simulink model "NeuromuscularModel3D"  (R2019b)
settings: Solver=ode15s  StartTime=0.0  StopTime=30  MaxStep=.01  RelTol=1e-4  AbsTol=1e-6  EnableMultiTasking=on
values from neighbouring files (symbols this model uses):
  dt_visual = 1/1000    (= 0.001)    [demorun.m]    (also in evaluateCost.m = 0.0333333333333; optimize.m = 0.0333333333333; optimize_Conly.m = 0.0333333333333; setVars.m = 0.0333333333333)
  initialTargetAngle = 70*pi/180    (= 1.2217304764)    [setInit.m]
  initialTargetAngleR = 90*pi/180    (= 1.57079632679)    [setInit.m]
  LongDelay = 0.020    (= 0.02)    [ControlParams2.m]
  MidDelay = 0.010    (= 0.01)    [ControlParams2.m]
  N = 82    [vcmaes_1.5cm_0.9ms_Umb10_kneelim1_mstoptorque2.mat]
  PreStimBFSHst = Gains(66)    [assignGains.m]    (also in assignGainsSagittal.m = GainsSagittal(51))
  PreStimBFSHsw = Gains(77)    [assignGains.m]    (also in assignGainsSagittal.m = GainsSagittal(60))
  PreStimGASst = Gains(67)    [assignGains.m]    (also in assignGainsSagittal.m = GainsSagittal(52))
  PreStimGASsw = Gains(78)    [assignGains.m]    (also in assignGainsSagittal.m = GainsSagittal(61))
  PreStimGLUst = Gains(62)    [assignGains.m]    (also in assignGainsSagittal.m = GainsSagittal(47))
  PreStimGLUsw = Gains(73)    [assignGains.m]    (also in assignGainsSagittal.m = GainsSagittal(56))
  PreStimHABst = Gains(70)    [assignGains.m]    (also in assignGainsCoronal.m = GainsCoronal(15))
  PreStimHABsw = Gains(81)    [assignGains.m]    (also in assignGainsCoronal.m = GainsCoronal(17))
  PreStimHADst = Gains(71)    [assignGains.m]    (also in assignGainsCoronal.m = GainsCoronal(16))
  PreStimHADsw = Gains(82)    [assignGains.m]    (also in assignGainsCoronal.m = GainsCoronal(18))
  PreStimHAMst = Gains(63)    [assignGains.m]    (also in assignGainsSagittal.m = GainsSagittal(48))
  PreStimHAMsw = Gains(74)    [assignGains.m]    (also in assignGainsSagittal.m = GainsSagittal(57))
  PreStimHFLst = Gains(61)    [assignGains.m]    (also in assignGainsSagittal.m = GainsSagittal(46))
  PreStimHFLsw = Gains(72)    [assignGains.m]    (also in assignGainsSagittal.m = GainsSagittal(55))
  PreStimRFst = Gains(64)    [assignGains.m]    (also in assignGainsSagittal.m = GainsSagittal(49))
  PreStimRFsw = Gains(75)    [assignGains.m]    (also in assignGainsSagittal.m = GainsSagittal(58))
  PreStimSOLst = Gains(68)    [assignGains.m]    (also in assignGainsSagittal.m = GainsSagittal(53))
  PreStimSOLsw = Gains(79)    [assignGains.m]    (also in assignGainsSagittal.m = GainsSagittal(62))
  PreStimTAst = Gains(69)    [assignGains.m]    (also in assignGainsSagittal.m = GainsSagittal(54))
  PreStimTAsw = Gains(80)    [assignGains.m]    (also in assignGainsSagittal.m = GainsSagittal(63))
  PreStimVASst = Gains(65)    [assignGains.m]    (also in assignGainsSagittal.m = GainsSagittal(50))
  PreStimVASsw = Gains(76)    [assignGains.m]    (also in assignGainsSagittal.m = GainsSagittal(59))
  ShortDelay = 0.005    [ControlParams2.m]
  simbiconGainD = 5*pi/180    (= 0.0872664625997)    [ControlParams2.m]    (also in assignGains.m = Gains(50); assignGains2.m = Gains(21); assignGainsSagittal.m = GainsSagittal(41))
  simbiconGainD_C = Gains(55)    [assignGains.m]    (also in assignGainsCoronal.m = GainsCoronal(11))
  simbiconGainV = 5*pi/180    (= 0.0872664625997)    [ControlParams2.m]    (also in assignGains.m = Gains(51); assignGains2.m = Gains(22); assignGainsSagittal.m = GainsSagittal(42))
  simbiconGainV_C = Gains(56)    [assignGains.m]    (also in assignGainsCoronal.m = GainsCoronal(12))
  simbiconLegAngle0 = 85*pi/180    (= 1.4835298642)    [ControlParams2.m]    (also in assignGains.m = Gains(49); assignGains2.m = Gains(23); assignGainsSagittal.m = GainsSagittal(40))
  simbiconLegAngle0_C = Gains(54)    [assignGains.m]    (also in assignGainsCoronal.m = GainsCoronal(10))
  vy0 = paramIC(10)*.2    [setInit.m]
  y0 = hatLeftHipToCenterDistWidth    [setInit.m]
undefined symbols (not defined in the file or in its folder): g, hatLeftHipToCenterDistWidth, hatLeftHipToCG, LongLoopDelay, magnitude, termination_height, thetaHATref, X, Y, Z
libraries: NeuroMuscularLibrary x120, nesl_utility x25, sm_lib x13, simulink x3
(part 1 of 3)
settings Model: ParamWorkspaceSource=ReferencedWorkspace  ExtModeTrigDuration=100  TunableVars=GainGAS,GainGLU,GainHAM,GainKneeOverExt,GainSOL,GainSOLTA,GainTA,GainVAS,Kglu,PosGainGG,SpeedGainGG,groundTheta,groundX,groundZ,hipDGain,hipPGain,kneeExtendGain,kneeFlexGain,kneeHoldGain1,kneeHoldGain2,kneeStopGain,legAngleFilter,legLengthClr,simbiconGainD,simbiconGainV,simbiconLegAngle0  TunableVarsStorageClass=Auto,Auto,Auto,Auto,Auto,Auto,Auto,Auto,Auto,Auto,Auto,Auto,Auto,Auto,Auto,Auto,Auto,Auto,Auto,Auto,Auto,Auto,Auto,Auto,Auto,Auto  TunableVarsTypeQualifier=,,,,,,,,,,,,,,,,,,,,,,,,,  Creator=nitisht  LastModifiedBy=Nathan
settings SolverCC: AutoScaleAbsTol=off  ZeroCrossAlgorithm=Adaptive
settings DataIOCC: LimitDataPoints=on  SaveFinalState=on  SaveFormat=StructureWithTime  SaveOutput=off  SaveState=on  ReturnWorkspaceOutputs=off  StateSaveName=tmp_raccel_xout  SignalLoggingName=tmp_raccel_logsout
settings OptimizationCC: DefaultParameterBehavior=Inlined  EfficientMapNaN2IntZero=off  LifeSpan=inf  SimCompilerOptimization=on  AccelVerboseBuild=on
settings DebuggingCC: SaveWithDisabledLinksMsg=none  UnderspecifiedInitializationDetection=Classic  MergeDetectMultiDrivingBlocksExec=none  IgnoredZcDiagnostic=none  SolverPrmCheckMsg=warning  StateNameClashWarn=warning  SFUnexpectedBacktrackingDiag=warning  SFNoUnconditionalDefaultTransitionDiag=warning  SFExecutionAtInitializationDiag=none  ArithmeticOperatorsInVariantConditions=warning
settings HardwareCC: ProdBitPerPointer=32  ProdBitPerSizeT=32  ProdBitPerPtrDiffT=32  ProdLargestAtomicFloat=None  ProdIntDivRoundTo=Undefined  ProdEndianess=Unspecified  ProdWordSize=32  ProdHWDeviceType=Generic->Unspecified (assume 32-bit Generic)  TargetBitPerPointer=64  TargetBitPerSizeT=64  TargetBitPerPtrDiffT=64  TargetLongLongMode=on  TargetIntDivRoundTo=Zero  TargetEndianess=LittleEndian  TargetWordSize=64  TargetHWDeviceType=MATLAB Host  ProdEqTarget=off
settings ModelReferenceCC: PropagateSignalLabelsOutOfModel=off
settings SFSimCC: SFSimEcho=off  SimUseLocalCustomCode=off  CustomCodeUndefinedFunction=UseInterfaceOnly
settings RTWCC: SystemTargetFile=raccel.tlc  TemplateMakefile=raccel_default_tmf  RTWUseLocalCustomCode=off  RTWUseSimCustomCode=on
settings CodeAppCC: GenerateComments=off  MaxIdLength=128  MangleLength=10  SimulinkBlockComments=off
settings RaccelTargetCC: GeneratePreprocessorConditionals=Disable all  MultiInstanceERTCode=off  PreserveStateflowLocalDataDimensions=off  ENABLE_SLEXEC_SSBRIDGE=0  RTWCAPIParams=off
settings ConfigComp: CovMetricSettings=dw  CovHtmlReporting=on  CovSaveCumulativeToWorkspaceVar=on  CovSaveSingleToWorkspaceVar=on  CovExternalEMLEnable=off  CovSFcnEnable=off
settings SimscapeCC: SimscapeNormalizeSystem=off
settings ConfigurationSet: Description=SimMechanics 2G

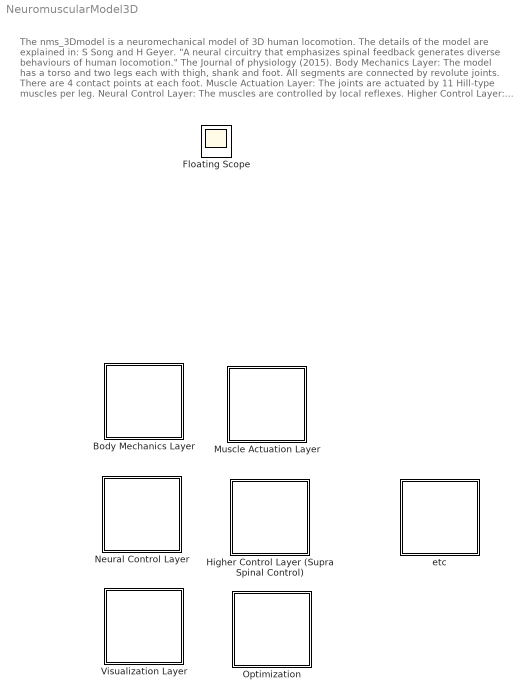
== system NeuromuscularModel3D ==
  note: The nms_3Dmodel is a neuromechanical model of 3D human locomotion.
      | The details of the model are explained in:
      | S Song and H Geyer. "A neural circuitry that emphasizes spinal feedback
      | generates diverse behaviours of human locomotion." The Journal of physiology (2015).
      |
      | Body Mechanics Layer:
      | The model has a torso and two legs each with thigh, shank and foot.
      | All segments are connected by revolute joints.
      | There are 4 contact points at each foot.
      |
      | Muscle Actuation Layer:
      | The joints are actuated by 11 Hill-type muscles per leg.
      |
      | Neural Control Layer:
      | The muscles are controlled by local reflexes.
      |
      | Higher Control Layer:
      | The reflex pathways are modulated by the higher layer control.
  Body Mechanics Layer : Subsystem
  Higher Control Layer (Supra Spinal Control) : Subsystem
  Muscle Actuation Layer : Subsystem
  Neural Control Layer : Subsystem
  Optimization : Subsystem
  Visualization Layer : Subsystem
  etc : Subsystem
  Floating Scope : Scope

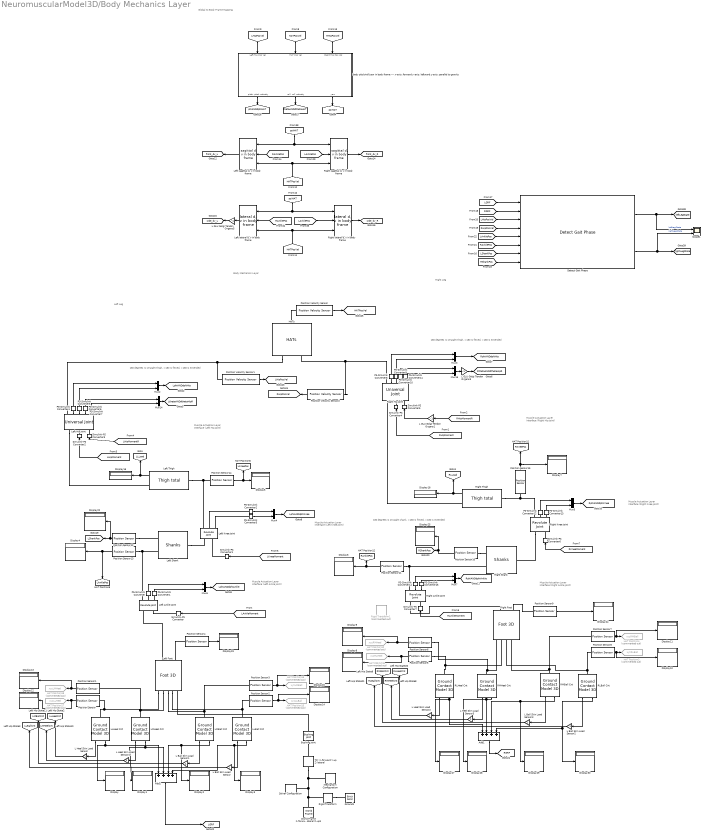
== system NeuromuscularModel3D/Body Mechanics Layer ==
  note: 180 degrees is straight thigh, <180 is flexed, >180 is extended
  note: Body Mechanics Layer
  note: Left Leg
  note: Right Leg
  note: Muscle Actuation
      | Layer Interface
      | (Left Hip Joint)
  note: Muscle Actuation
      | Layer Interface
      | (Left Knee Joint)
  note: Muscle Actuation
      | Layer Interface
      | (Left Ankle Joint)
  note: Muscle Actuation
      | Layer Interface
      | (Right Ankle Joint)
  note: Muscle Actuation
      | Layer Interface
      | (Right Knee Joint)
  note: Muscle Actuation
      | Layer Interface
      | (Right Hip Joint)
  note: Global to Body Frame Mapping
  note: 180 degrees is straight thigh, <180 is flexed, >180 is extended
  note: 180 degrees is straight shank, <180 is flexed, >180 is extended
  Add1 : Sum  Inputs=4
  Add2 : Sum  Inputs=4
  Bushing Joint : sm_lib/Joints/Bushing Joint  JointMode=Normal  SenseConstraintForce=off  SenseConstraintForceX=off  SenseConstraintForceY=off  SenseConstraintForceZ=off  SenseConstraintTorque=off  SenseConstraintTorqueX=off  SenseConstraintTorqueY=off  SenseConstraintTorqueZ=off  SenseTotalForce=off  SenseTotalForceX=off  SenseTotalForceY=off  SenseTotalForceZ=off  SenseTotalTorque=off  SenseTotalTorqueX=off  SenseTotalTorqueY=off  SenseTotalTorqueZ=off  CompositeWrenchDir=FollowerOnBase  CompositeWrenchFrame=BaseFrame  PxEquilibriumPosition=0  PxEquilibriumPositionUnits=m  PxSpringStiffness=0  PxSpringStiffnessUnits=N/m  PxDampingCoefficient=0  PxDampingCoefficientUnits=N/(m/s)  PxTorqueActuationMode=NoTorque  PxMotionActuationMode=ComputedMotion  PxSensePosition=off  PxSenseVelocity=off  PxSenseAcceleration=off  PxSenseTorqueForce=off  PxSenseLowerLimitTorqueForce=off  PxSenseUpperLimitTorqueForce=off  PxLowerLimitSpecify=off  PxLowerLimitBound=-1  PxLowerLimitBoundUnits=m  PxLowerLimitStiffness=1e6  PxLowerLimitStiffnessUnits=N/m  PxLowerLimitDamping=1e3  PxLowerLimitDampingUnits=N/(m/s)  PxLowerLimitTransitionRegionWidth=1e-4  PxLowerLimitTransitionRegionWidthUnits=m  PxUpperLimitSpecify=off  PxUpperLimitBound=1  PxUpperLimitBoundUnits=m  PxUpperLimitStiffness=1e6  PxUpperLimitStiffnessUnits=N/m  PxUpperLimitDamping=1e3  PxUpperLimitDampingUnits=N/(m/s)  PxUpperLimitTransitionRegionWidth=1e-4  PxUpperLimitTransitionRegionWidthUnits=m  PxPositionTargetSpecify=on  PxPositionTargetPriority=High  PxPositionTargetValue=x0  PxPositionTargetValueUnits=m  PxVelocityTargetSpecify=on  PxVelocityTargetPriority=High  PxVelocityTargetValue=vx0  PxVelocityTargetValueUnits=m/s  PyEquilibriumPosition=0  PyEquilibriumPositionUnits=m  PySpringStiffness=0  PySpringStiffnessUnits=N/m  PyDampingCoefficient=0  PyDampingCoefficientUnits=N/(m/s)  PyTorqueActuationMode=NoTorque  PyMotionActuationMode=ComputedMotion  PySensePosition=off  PySenseVelocity=off  PySenseAcceleration=off  PySenseTorqueForce=off  PySenseLowerLimitTorqueForce=off  PySenseUpperLimitTorqueForce=off  PyLowerLimitSpecify=off  PyLowerLimitBound=-1  PyLowerLimitBoundUnits=m  PyLowerLimitStiffness=1e6  PyLowerLimitStiffnessUnits=N/m  PyLowerLimitDamping=1e3  PyLowerLimitDampingUnits=N/(m/s)  PyLowerLimitTransitionRegionWidth=1e-4  PyLowerLimitTransitionRegionWidthUnits=m  PyUpperLimitSpecify=off  PyUpperLimitBound=1  PyUpperLimitBoundUnits=m  PyUpperLimitStiffness=1e6  PyUpperLimitStiffnessUnits=N/m  PyUpperLimitDamping=1e3  PyUpperLimitDampingUnits=N/(m/s)  PyUpperLimitTransitionRegionWidth=1e-4  PyUpperLimitTransitionRegionWidthUnits=m  PyPositionTargetSpecify=on  PyPositionTargetPriority=High  PyPositionTargetValue=z0  PyPositionTargetValueUnits=m  PyVelocityTargetSpecify=on  PyVelocityTargetPriority=High  PyVelocityTargetValue=0  PyVelocityTargetValueUnits=m/s  PzEquilibriumPosition=0  PzEquilibriumPositionUnits=m  PzSpringStiffness=0  PzSpringStiffnessUnits=N/m  PzDampingCoefficient=0  PzDampingCoefficientUnits=N/(m/s)  PzTorqueActuationMode=NoTorque  PzMotionActuationMode=ComputedMotion  PzSensePosition=off  PzSenseVelocity=off  PzSenseAcceleration=off  PzSenseTorqueForce=off  PzSenseLowerLimitTorqueForce=off  PzSenseUpperLimitTorqueForce=off  PzLowerLimitSpecify=off  PzLowerLimitBound=-1  PzLowerLimitBoundUnits=m  PzLowerLimitStiffness=1e6  PzLowerLimitStiffnessUnits=N/m  PzLowerLimitDamping=1e3  PzLowerLimitDampingUnits=N/(m/s)  PzLowerLimitTransitionRegionWidth=1e-4  PzLowerLimitTransitionRegionWidthUnits=m  PzUpperLimitSpecify=off  PzUpperLimitBound=1  PzUpperLimitBoundUnits=m  PzUpperLimitStiffness=1e6  PzUpperLimitStiffnessUnits=N/m  PzUpperLimitDamping=1e3  PzUpperLimitDampingUnits=N/(m/s)  PzUpperLimitTransitionRegionWidth=1e-4  PzUpperLimitTransitionRegionWidthUnits=m  PzPositionTargetSpecify=on  PzPositionTargetPriority=High  PzPositionTargetValue=-y0  PzPositionTargetValueUnits=m  PzVelocityTargetSpecify=on  PzVelocityTargetPriority=High  PzVelocityTargetValue=-vy0  PzVelocityTargetValueUnits=m/s  RxEquilibriumPosition=0  RxEquilibriumPositionUnits=deg  RxSpringStiffness=0  RxSpringStiffnessUnits=N*m/deg  RxDampingCoefficient=0  RxDampingCoefficientUnits=N*m/(deg/s)  RxTorqueActuationMode=NoTorque  RxMotionActuationMode=ComputedMotion  RxSensePosition=off  RxSenseVelocity=off  RxSenseAcceleration=off  RxSenseTorqueForce=off  RxSenseLowerLimitTorqueForce=off  RxSenseUpperLimitTorqueForce=off  RxLowerLimitSpecify=off  RxLowerLimitBound=-90  RxLowerLimitBoundUnits=deg  RxLowerLimitStiffness=1e4  RxLowerLimitStiffnessUnits=N*m/deg  RxLowerLimitDamping=10  RxLowerLimitDampingUnits=N*m/(deg/s)  RxLowerLimitTransitionRegionWidth=0.1  RxLowerLimitTransitionRegionWidthUnits=deg  RxUpperLimitSpecify=off  RxUpperLimitBound=90  RxUpperLimitBoundUnits=deg  RxUpperLimitStiffness=1e4  RxUpperLimitStiffnessUnits=N*m/deg  RxUpperLimitDamping=10  RxUpperLimitDampingUnits=N*m/(deg/s)  RxUpperLimitTransitionRegionWidth=0.1  RxUpperLimitTransitionRegionWidthUnits=deg  RxPositionTargetSpecify=on  RxPositionTargetPriority=High  RxPositionTargetValue=roll0  RxPositionTargetValueUnits=rad  RxVelocityTargetSpecify=on  RxVelocityTargetPriority=High  RxVelocityTargetValue=0  RxVelocityTargetValueUnits=rad/s  RyEquilibriumPosition=0  RyEquilibriumPositionUnits=deg  RySpringStiffness=0  RySpringStiffnessUnits=N*m/deg  RyDampingCoefficient=0  RyDampingCoefficientUnits=N*m/(deg/s)  RyTorqueActuationMode=NoTorque  RyMotionActuationMode=ComputedMotion  RySensePosition=off  RySenseVelocity=off  RySenseAcceleration=off  RySenseTorqueForce=off  RySenseLowerLimitTorqueForce=off  RySenseUpperLimitTorqueForce=off  RyLowerLimitSpecify=off  RyLowerLimitBound=-90  RyLowerLimitBoundUnits=deg  RyLowerLimitStiffness=1e4  RyLowerLimitStiffnessUnits=N*m/deg  RyLowerLimitDamping=10  RyLowerLimitDampingUnits=N*m/(deg/s)  RyLowerLimitTransitionRegionWidth=0.1  RyLowerLimitTransitionRegionWidthUnits=deg  RyUpperLimitSpecify=off  RyUpperLimitBound=90  RyUpperLimitBoundUnits=deg  RyUpperLimitStiffness=1e4  RyUpperLimitStiffnessUnits=N*m/deg  RyUpperLimitDamping=10  RyUpperLimitDampingUnits=N*m/(deg/s)  RyUpperLimitTransitionRegionWidth=0.1  RyUpperLimitTransitionRegionWidthUnits=deg  RyPositionTargetSpecify=on  RyPositionTargetPriority=High  RyPositionTargetValue=yaw0  RyPositionTargetValueUnits=rad  RyVelocityTargetSpecify=on  RyVelocityTargetPriority=High  RyVelocityTargetValue=0  RyVelocityTargetValueUnits=rad/s  RzEquilibriumPosition=0  RzEquilibriumPositionUnits=deg  RzSpringStiffness=0  RzSpringStiffnessUnits=N*m/deg  RzDampingCoefficient=0  RzDampingCoefficientUnits=N*m/(deg/s)  RzTorqueActuationMode=NoTorque  RzMotionActuationMode=ComputedMotion  RzSensePosition=off  RzSenseVelocity=off  RzSenseAcceleration=off  RzSenseTorqueForce=off  RzSenseLowerLimitTorqueForce=off  RzSenseUpperLimitTorqueForce=off  RzLowerLimitSpecify=off  RzLowerLimitBound=-90  RzLowerLimitBoundUnits=deg  RzLowerLimitStiffness=1e4  RzLowerLimitStiffnessUnits=N*m/deg  RzLowerLimitDamping=10  RzLowerLimitDampingUnits=N*m/(deg/s)  RzLowerLimitTransitionRegionWidth=0.1  RzLowerLimitTransitionRegionWidthUnits=deg  RzUpperLimitSpecify=off  RzUpperLimitBound=90  RzUpperLimitBoundUnits=deg  RzUpperLimitStiffness=1e4  RzUpperLimitStiffnessUnits=N*m/deg  RzUpperLimitDamping=10  RzUpperLimitDampingUnits=N*m/(deg/s)  RzUpperLimitTransitionRegionWidth=0.1  RzUpperLimitTransitionRegionWidthUnits=deg  RzPositionTargetSpecify=off  RzPositionTargetPriority=High  RzPositionTargetValue=0  RzPositionTargetValueUnits=deg  RzVelocityTargetSpecify=off  RzVelocityTargetPriority=High  RzVelocityTargetValue=0  RzVelocityTargetValueUnits=deg/s
      settings: SourceProductName=Simscape Multibody
  Detect Gait Phase : NeuroMuscularLibrary/Detect Gait Phase  SystemSampleTime=-1  Latency=0  AutoFrameSizeCalculation=off
  Display{,1..16,18,22..25,27..30} (26 alike) : Display
  Ground1 : sm_lib/Body Elements/Brick Solid  GraphicAmbientColor=[0.15 0.15 0.15 1.0]  BasedOnType=Density  BrickDimensions=[3 1 .01]  BrickDimensionUnits=m  CenterOfMass=[0 0 0]  CenterOfMassUnits=m  GraphicDiffuseColor=[0.4 0.2 0.0]  Density=1000  DensityUnits=kg/(m^3)  DoExposeReferenceFrame=on  GraphicEmissiveColor=[0.0 0.0 0.0 1.0]  ExportEntireGeometry=off  SerializedFrames=<Frames/>  MarkerShape=Sphere  MarkerSize=10  GraphicType=FromGeometry  InertiaType=Custom  Mass=0  MassUnits=kg  MomentsOfInertia=[0 0 0]  MomentsOfInertiaUnits=kg*m^2  GraphicOpacity=1.0  ProductsOfInertia=[0 0 0]  ProductsOfInertiaUnits=kg*m^2  GraphicShininess=75  GraphicSpecularColor=[0.5 0.5 0.5 1.0]  GraphicVisPropType=SimpleVisualProperties
  HAT Position10 : Goto  Commented=on  GotoTag=xyzRMHeel  TagVisibility=global
  HAT Position15 : Goto  Commented=on  GotoTag=xyzLLBall  TagVisibility=global
  HAT Position16 : Goto  Commented=on  GotoTag=xyzLMBall  TagVisibility=global
  HAT Position17 : Goto  Commented=on  GotoTag=xyzLLHeel  TagVisibility=global
  HAT Position18 : Goto  Commented=on  GotoTag=xyzLMHeel  TagVisibility=global
  HAT Position3 : Goto  Commented=on  GotoTag=xyzRLBall  TagVisibility=global
  HAT Position4 : Goto  Commented=on  GotoTag=xyzRMBall  TagVisibility=global
  HAT Position9 : Goto  Commented=on  GotoTag=xyzRLHeel  TagVisibility=global
  HATs : NeuroMuscularLibrary/HATs  SystemSampleTime=-1  Latency=0  AutoFrameSizeCalculation=off
  L Ball Skin Load Sensor{,1..3} (4 alike) : Gain
  L GLU Golgi Tendon Organs1 : Gain  Gain=-1
  L GLU Golgi Tendon Organs3 : Gain  Gain=-1
  L GLU Golgi Tendon Organs5 : Gain  Gain=-1
  L Heel Skin Load Sensor{,1..3} (4 alike) : Gain
  LLBall Cnt : NeuroMuscularLibrary/Ground Contact Model 3D  SystemSampleTime=-1  Latency=0  AutoFrameSizeCalculation=off
  LLHeel Cnt : NeuroMuscularLibrary/Ground Contact Model 3D  SystemSampleTime=-1  Latency=0  AutoFrameSizeCalculation=off
  LMBall Cnt : NeuroMuscularLibrary/Ground Contact Model 3D  SystemSampleTime=-1  Latency=0  AutoFrameSizeCalculation=off
  LMHeel Cnt : NeuroMuscularLibrary/Ground Contact Model 3D  SystemSampleTime=-1  Latency=0  AutoFrameSizeCalculation=off
  Left Knee Joint : sm_lib/Joints/Revolute Joint  JointMode=Normal  SenseConstraintForce=off  SenseConstraintForceX=off  SenseConstraintForceY=off  SenseConstraintForceZ=off  SenseConstraintTorque=off  SenseConstraintTorqueX=off  SenseConstraintTorqueY=off  SenseConstraintTorqueZ=off  SenseTotalForce=off  SenseTotalForceX=off  SenseTotalForceY=off  SenseTotalForceZ=off  SenseTotalTorque=off  SenseTotalTorqueX=off  SenseTotalTorqueY=off  SenseTotalTorqueZ=off  CompositeWrenchDir=FollowerOnBase  CompositeWrenchFrame=BaseFrame  EquilibriumPosition=0  EquilibriumPositionUnits=deg  SpringStiffness=0  SpringStiffnessUnits=N*m/deg  DampingCoefficient=0  DampingCoefficientUnits=N*m/(deg/s)  TorqueActuationMode=InputTorque  MotionActuationMode=ComputedMotion  SensePosition=on  SenseVelocity=on  SenseAcceleration=off  SenseTorqueForce=off  SenseLowerLimitTorqueForce=off  SenseUpperLimitTorqueForce=off  LowerLimitSpecify=off  LowerLimitBound=-90  LowerLimitBoundUnits=deg  LowerLimitStiffness=1e4  LowerLimitStiffnessUnits=N*m/deg  LowerLimitDamping=10  LowerLimitDampingUnits=N*m/(deg/s)  LowerLimitTransitionRegionWidth=0.1  LowerLimitTransitionRegionWidthUnits=deg  UpperLimitSpecify=off  UpperLimitBound=90  UpperLimitBoundUnits=deg  UpperLimitStiffness=1e4  UpperLimitStiffnessUnits=N*m/deg  UpperLimitDamping=10  UpperLimitDampingUnits=N*m/(deg/s)  UpperLimitTransitionRegionWidth=0.1  UpperLimitTransitionRegionWidthUnits=deg  PositionTargetSpecify=on  PositionTargetPriority=High  PositionTargetValue=LphiKnee0  PositionTargetValueUnits=rad  VelocityTargetSpecify=on  VelocityTargetPriority=High  VelocityTargetValue=0  VelocityTargetValueUnits=rad/s
  Left Ankle joint : sm_lib/Joints/Revolute Joint  JointMode=Normal  SenseConstraintForce=off  SenseConstraintForceX=off  SenseConstraintForceY=off  SenseConstraintForceZ=off  SenseConstraintTorque=off  SenseConstraintTorqueX=off  SenseConstraintTorqueY=off  SenseConstraintTorqueZ=off  SenseTotalForce=off  SenseTotalForceX=off  SenseTotalForceY=off  SenseTotalForceZ=off  SenseTotalTorque=off  SenseTotalTorqueX=off  SenseTotalTorqueY=off  SenseTotalTorqueZ=off  CompositeWrenchDir=FollowerOnBase  CompositeWrenchFrame=BaseFrame  EquilibriumPosition=0  EquilibriumPositionUnits=deg  SpringStiffness=0  SpringStiffnessUnits=N*m/deg  DampingCoefficient=0  DampingCoefficientUnits=N*m/(deg/s)  TorqueActuationMode=InputTorque  MotionActuationMode=ComputedMotion  SensePosition=on  SenseVelocity=on  SenseAcceleration=off  SenseTorqueForce=off  SenseLowerLimitTorqueForce=off  SenseUpperLimitTorqueForce=off  LowerLimitSpecify=off  LowerLimitBound=-90  LowerLimitBoundUnits=deg  LowerLimitStiffness=1e4  LowerLimitStiffnessUnits=N*m/deg  LowerLimitDamping=10  LowerLimitDampingUnits=N*m/(deg/s)  LowerLimitTransitionRegionWidth=0.1  LowerLimitTransitionRegionWidthUnits=deg  UpperLimitSpecify=off  UpperLimitBound=90  UpperLimitBoundUnits=deg  UpperLimitStiffness=1e4  UpperLimitStiffnessUnits=N*m/deg  UpperLimitDamping=10  UpperLimitDampingUnits=N*m/(deg/s)  UpperLimitTransitionRegionWidth=0.1  UpperLimitTransitionRegionWidthUnits=deg  PositionTargetSpecify=on  PositionTargetPriority=High  PositionTargetValue=LphiAnkle0  PositionTargetValueUnits=rad  VelocityTargetSpecify=on  VelocityTargetPriority=High  VelocityTargetValue=0  VelocityTargetValueUnits=rad/s
  Left Foot : NeuroMuscularLibrary/Foot 3D  SystemSampleTime=-1  Latency=0  AutoFrameSizeCalculation=off
  Left Hip Joint : sm_lib/Joints/Universal Joint  JointMode=Normal  SenseConstraintForce=off  SenseConstraintForceX=off  SenseConstraintForceY=off  SenseConstraintForceZ=off  SenseConstraintTorque=off  SenseConstraintTorqueX=off  SenseConstraintTorqueY=off  SenseConstraintTorqueZ=off  SenseTotalForce=off  SenseTotalForceX=off  SenseTotalForceY=off  SenseTotalForceZ=off  SenseTotalTorque=off  SenseTotalTorqueX=off  SenseTotalTorqueY=off  SenseTotalTorqueZ=off  CompositeWrenchDir=FollowerOnBase  CompositeWrenchFrame=BaseFrame  RxEquilibriumPosition=0  RxEquilibriumPositionUnits=deg  RxSpringStiffness=0  RxSpringStiffnessUnits=N*m/deg  RxDampingCoefficient=0  RxDampingCoefficientUnits=N*m/(deg/s)  RxTorqueActuationMode=InputTorque  RxMotionActuationMode=ComputedMotion  RxSensePosition=on  RxSenseVelocity=on  RxSenseAcceleration=off  RxSenseTorqueForce=off  RxSenseLowerLimitTorqueForce=off  RxSenseUpperLimitTorqueForce=off  RxLowerLimitSpecify=off  RxLowerLimitBound=-90  RxLowerLimitBoundUnits=deg  RxLowerLimitStiffness=1e4  RxLowerLimitStiffnessUnits=N*m/deg  RxLowerLimitDamping=10  RxLowerLimitDampingUnits=N*m/(deg/s)  RxLowerLimitTransitionRegionWidth=0.1  RxLowerLimitTransitionRegionWidthUnits=deg  RxUpperLimitSpecify=off  RxUpperLimitBound=90  RxUpperLimitBoundUnits=deg  RxUpperLimitStiffness=1e4  RxUpperLimitStiffnessUnits=N*m/deg  RxUpperLimitDamping=10  RxUpperLimitDampingUnits=N*m/(deg/s)  RxUpperLimitTransitionRegionWidth=0.1  RxUpperLimitTransitionRegionWidthUnits=deg  RxPositionTargetSpecify=on  RxPositionTargetPriority=High  RxPositionTargetValue=LphiHip0  RxPositionTargetValueUnits=rad  RxVelocityTargetSpecify=on  RxVelocityTargetPriority=High  RxVelocityTargetValue=0  RxVelocityTargetValueUnits=rad/s  RyEquilibriumPosition=0  RyEquilibriumPositionUnits=deg  RySpringStiffness=0  RySpringStiffnessUnits=N*m/deg  RyDampingCoefficient=0  RyDampingCoefficientUnits=N*m/(deg/s)  RyTorqueActuationMode=InputTorque  RyMotionActuationMode=ComputedMotion  RySensePosition=on  RySenseVelocity=on  RySenseAcceleration=off  RySenseTorqueForce=off  RySenseLowerLimitTorqueForce=off  RySenseUpperLimitTorqueForce=off  RyLowerLimitSpecify=off  RyLowerLimitBound=-90  RyLowerLimitBoundUnits=deg  RyLowerLimitStiffness=1e4  RyLowerLimitStiffnessUnits=N*m/deg  RyLowerLimitDamping=10  RyLowerLimitDampingUnits=N*m/(deg/s)  RyLowerLimitTransitionRegionWidth=0.1  RyLowerLimitTransitionRegionWidthUnits=deg  RyUpperLimitSpecify=off  RyUpperLimitBound=90  RyUpperLimitBoundUnits=deg  RyUpperLimitStiffness=1e4  RyUpperLimitStiffnessUnits=N*m/deg  RyUpperLimitDamping=10  RyUpperLimitDampingUnits=N*m/(deg/s)  RyUpperLimitTransitionRegionWidth=0.1  RyUpperLimitTransitionRegionWidthUnits=deg  RyPositionTargetSpecify=on  RyPositionTargetPriority=High  RyPositionTargetValue=LphiHipR0  RyPositionTargetValueUnits=rad  RyVelocityTargetSpecify=on  RyVelocityTargetPriority=High  RyVelocityTargetValue=0  RyVelocityTargetValueUnits=rad/s
      settings: SourceProductName=Simscape Multibody
  Left Shank : NeuroMuscularLibrary/Shanks  SystemSampleTime=-1  Latency=0  AutoFrameSizeCalculation=off
      link override To CG: RotationMethod=None  BaseAlignAxisA=+Z  BaseAlignAxisB=+Y
  Left Thigh : NeuroMuscularLibrary/Thigh total  SystemSampleTime=-1  Latency=0  AutoFrameSizeCalculation=off
  "Left lateral d, v in body frame" : NeuroMuscularLibrary/lateral d, v in body frame  SystemSampleTime=-1  Latency=0  AutoFrameSizeCalculation=off
      link override Selector3: InputPortWidth=6
  "Left sagittal d, v in body frame" : NeuroMuscularLibrary/sagittal d, v in body frame  SystemSampleTime=-1  Latency=0  AutoFrameSizeCalculation=off
  Mechanism Configuration : sm_lib/Utilities/Mechanism Configuration  UniformGravity=Constant  GravityVector=[0 0 -g]  GravityUnits=m/s^2  LinearizationDelta=0.001
  Mux{2..7,14..15} (8 alike) : Mux  Inputs=2
  PS-Simulink Converter{,2,4,6,8,10,12,14} (8 alike) : nesl_utility/PS-Simulink Converter  PhysicalDomain=network_engine_domain  SubClassName=ps_output  LeftPortType=input  RightPortType=output  PseudoPeriodic=off  Frequencies=[]  Unit=rad  AffineConversion=off
  PS-Simulink Converter{1,3,5,7,9,11,13,15} (8 alike) : nesl_utility/PS-Simulink Converter  PhysicalDomain=network_engine_domain  SubClassName=ps_output  LeftPortType=input  RightPortType=output  PseudoPeriodic=off  Frequencies=[]  Unit=rad/s  AffineConversion=off
  Position Sensor{,1..15} (16 alike) : NeuroMuscularLibrary/Position Sensor  SystemSampleTime=-1  Latency=0  AutoFrameSizeCalculation=off
  Position Velocity Sensor : NeuroMuscularLibrary/Position Velocity Sensor  SystemSampleTime=-1  Latency=0  AutoFrameSizeCalculation=off
  Position Velocity Sensor1 : NeuroMuscularLibrary/Position Velocity Sensor  SystemSampleTime=-1  Latency=0  AutoFrameSizeCalculation=off
  Position Velocity Sensor2 : NeuroMuscularLibrary/Position Velocity Sensor  SystemSampleTime=-1  Latency=0  AutoFrameSizeCalculation=off
  RLBall Cnt : NeuroMuscularLibrary/Ground Contact Model 3D  SystemSampleTime=-1  Latency=0  AutoFrameSizeCalculation=off
  RLHeel Cnt : NeuroMuscularLibrary/Ground Contact Model 3D  SystemSampleTime=-1  Latency=0  AutoFrameSizeCalculation=off
  RMBall Cnt : NeuroMuscularLibrary/Ground Contact Model 3D  SystemSampleTime=-1  Latency=0  AutoFrameSizeCalculation=off
  "RMHeel Cnt " : NeuroMuscularLibrary/Ground Contact Model 3D  SystemSampleTime=-1  Latency=0  AutoFrameSizeCalculation=off
  Right Ankle Joint : sm_lib/Joints/Revolute Joint  JointMode=Normal  SenseConstraintForce=off  SenseConstraintForceX=off  SenseConstraintForceY=off  SenseConstraintForceZ=off  SenseConstraintTorque=off  SenseConstraintTorqueX=off  SenseConstraintTorqueY=off  SenseConstraintTorqueZ=off  SenseTotalForce=off  SenseTotalForceX=off  SenseTotalForceY=off  SenseTotalForceZ=off  SenseTotalTorque=off  SenseTotalTorqueX=off  SenseTotalTorqueY=off  SenseTotalTorqueZ=off  CompositeWrenchDir=FollowerOnBase  CompositeWrenchFrame=BaseFrame  EquilibriumPosition=0  EquilibriumPositionUnits=deg  SpringStiffness=0  SpringStiffnessUnits=N*m/deg  DampingCoefficient=0  DampingCoefficientUnits=N*m/(deg/s)  TorqueActuationMode=InputTorque  MotionActuationMode=ComputedMotion  SensePosition=on  SenseVelocity=on  SenseAcceleration=off  SenseTorqueForce=off  SenseLowerLimitTorqueForce=off  SenseUpperLimitTorqueForce=off  LowerLimitSpecify=off  LowerLimitBound=-90  LowerLimitBoundUnits=deg  LowerLimitStiffness=1e4  LowerLimitStiffnessUnits=N*m/deg  LowerLimitDamping=10  LowerLimitDampingUnits=N*m/(deg/s)  LowerLimitTransitionRegionWidth=0.1  LowerLimitTransitionRegionWidthUnits=deg  UpperLimitSpecify=off  UpperLimitBound=90  UpperLimitBoundUnits=deg  UpperLimitStiffness=1e4  UpperLimitStiffnessUnits=N*m/deg  UpperLimitDamping=10  UpperLimitDampingUnits=N*m/(deg/s)  UpperLimitTransitionRegionWidth=0.1  UpperLimitTransitionRegionWidthUnits=deg  PositionTargetSpecify=on  PositionTargetPriority=High  PositionTargetValue=RphiAnkle0  PositionTargetValueUnits=rad  VelocityTargetSpecify=on  VelocityTargetPriority=High  VelocityTargetValue=0  VelocityTargetValueUnits=rad/s
  Right Foot : NeuroMuscularLibrary/Foot 3D  SystemSampleTime=-1  Latency=0  AutoFrameSizeCalculation=off
  Right Hip joint : sm_lib/Joints/Universal Joint  JointMode=Normal  SenseConstraintForce=off  SenseConstraintForceX=off  SenseConstraintForceY=off  SenseConstraintForceZ=off  SenseConstraintTorque=off  SenseConstraintTorqueX=off  SenseConstraintTorqueY=off  SenseConstraintTorqueZ=off  SenseTotalForce=off  SenseTotalForceX=off  SenseTotalForceY=off  SenseTotalForceZ=off  SenseTotalTorque=off  SenseTotalTorqueX=off  SenseTotalTorqueY=off  SenseTotalTorqueZ=off  CompositeWrenchDir=FollowerOnBase  CompositeWrenchFrame=BaseFrame  RxEquilibriumPosition=0  RxEquilibriumPositionUnits=deg  RxSpringStiffness=0  RxSpringStiffnessUnits=N*m/deg  RxDampingCoefficient=0  RxDampingCoefficientUnits=N*m/(deg/s)  RxTorqueActuationMode=InputTorque  RxMotionActuationMode=ComputedMotion  RxSensePosition=on  RxSenseVelocity=on  RxSenseAcceleration=off  RxSenseTorqueForce=off  RxSenseLowerLimitTorqueForce=off  RxSenseUpperLimitTorqueForce=off  RxLowerLimitSpecify=off  RxLowerLimitBound=-90  RxLowerLimitBoundUnits=deg  RxLowerLimitStiffness=1e4  RxLowerLimitStiffnessUnits=N*m/deg  RxLowerLimitDamping=10  RxLowerLimitDampingUnits=N*m/(deg/s)  RxLowerLimitTransitionRegionWidth=0.1  RxLowerLimitTransitionRegionWidthUnits=deg  RxUpperLimitSpecify=off  RxUpperLimitBound=90  RxUpperLimitBoundUnits=deg  RxUpperLimitStiffness=1e4  RxUpperLimitStiffnessUnits=N*m/deg  RxUpperLimitDamping=10  RxUpperLimitDampingUnits=N*m/(deg/s)  RxUpperLimitTransitionRegionWidth=0.1  RxUpperLimitTransitionRegionWidthUnits=deg  RxPositionTargetSpecify=on  RxPositionTargetPriority=High  RxPositionTargetValue=RphiHip0  RxPositionTargetValueUnits=rad  RxVelocityTargetSpecify=on  RxVelocityTargetPriority=High  RxVelocityTargetValue=0  RxVelocityTargetValueUnits=rad/s  RyEquilibriumPosition=0  RyEquilibriumPositionUnits=deg  RySpringStiffness=0  RySpringStiffnessUnits=N*m/deg  RyDampingCoefficient=0  RyDampingCoefficientUnits=N*m/(deg/s)  RyTorqueActuationMode=InputTorque  RyMotionActuationMode=ComputedMotion  RySensePosition=on  RySenseVelocity=on  RySenseAcceleration=off  RySenseTorqueForce=off  RySenseLowerLimitTorqueForce=off  RySenseUpperLimitTorqueForce=off  RyLowerLimitSpecify=off  RyLowerLimitBound=-90  RyLowerLimitBoundUnits=deg  RyLowerLimitStiffness=1e4  RyLowerLimitStiffnessUnits=N*m/deg  RyLowerLimitDamping=10  RyLowerLimitDampingUnits=N*m/(deg/s)  RyLowerLimitTransitionRegionWidth=0.1  RyLowerLimitTransitionRegionWidthUnits=deg  RyUpperLimitSpecify=off  RyUpperLimitBound=90  RyUpperLimitBoundUnits=deg  RyUpperLimitStiffness=1e4  RyUpperLimitStiffnessUnits=N*m/deg  RyUpperLimitDamping=10  RyUpperLimitDampingUnits=N*m/(deg/s)  RyUpperLimitTransitionRegionWidth=0.1  RyUpperLimitTransitionRegionWidthUnits=deg  RyPositionTargetSpecify=on  RyPositionTargetPriority=High  RyPositionTargetValue=RphiHipR0  RyPositionTargetValueUnits=rad  RyVelocityTargetSpecify=on  RyVelocityTargetPriority=High  RyVelocityTargetValue=0  RyVelocityTargetValueUnits=rad/s
      settings: SourceProductName=Simscape Multibody
  Right Knee joint : sm_lib/Joints/Revolute Joint  JointMode=Normal  SenseConstraintForce=off  SenseConstraintForceX=off  SenseConstraintForceY=off  SenseConstraintForceZ=off  SenseConstraintTorque=off  SenseConstraintTorqueX=off  SenseConstraintTorqueY=off  SenseConstraintTorqueZ=off  SenseTotalForce=off  SenseTotalForceX=off  SenseTotalForceY=off  SenseTotalForceZ=off  SenseTotalTorque=off  SenseTotalTorqueX=off  SenseTotalTorqueY=off  SenseTotalTorqueZ=off  CompositeWrenchDir=FollowerOnBase  CompositeWrenchFrame=BaseFrame  EquilibriumPosition=0  EquilibriumPositionUnits=deg  SpringStiffness=0  SpringStiffnessUnits=N*m/deg  DampingCoefficient=0  DampingCoefficientUnits=N*m/(deg/s)  TorqueActuationMode=InputTorque  MotionActuationMode=ComputedMotion  SensePosition=on  SenseVelocity=on  SenseAcceleration=off  SenseTorqueForce=off  SenseLowerLimitTorqueForce=off  SenseUpperLimitTorqueForce=off  LowerLimitSpecify=off  LowerLimitBound=-90  LowerLimitBoundUnits=deg  LowerLimitStiffness=1e4  LowerLimitStiffnessUnits=N*m/deg  LowerLimitDamping=10  LowerLimitDampingUnits=N*m/(deg/s)  LowerLimitTransitionRegionWidth=0.1  LowerLimitTransitionRegionWidthUnits=deg  UpperLimitSpecify=off  UpperLimitBound=90  UpperLimitBoundUnits=deg  UpperLimitStiffness=1e4  UpperLimitStiffnessUnits=N*m/deg  UpperLimitDamping=10  UpperLimitDampingUnits=N*m/(deg/s)  UpperLimitTransitionRegionWidth=0.1  UpperLimitTransitionRegionWidthUnits=deg  PositionTargetSpecify=on  PositionTargetPriority=High  PositionTargetValue=RphiKnee0  PositionTargetValueUnits=rad  VelocityTargetSpecify=on  VelocityTargetPriority=High  VelocityTargetValue=0  VelocityTargetValueUnits=rad/s
  Right Shank : NeuroMuscularLibrary/Shanks  SystemSampleTime=-1  Latency=0  AutoFrameSizeCalculation=off
  Right Thigh : NeuroMuscularLibrary/Thigh total  SystemSampleTime=-1  Latency=0  AutoFrameSizeCalculation=off
  "Right lateral d, v in body frame" : NeuroMuscularLibrary/lateral d, v in body frame  SystemSampleTime=-1  Latency=0  AutoFrameSizeCalculation=off
  "Right sagittal d, v in body frame" : NeuroMuscularLibrary/sagittal d, v in body frame  SystemSampleTime=-1  Latency=0  AutoFrameSizeCalculation=off
  Rigid Transform1 : sm_lib/Frames and Transforms/Rigid Transform  Commented=on  TranslationMethod=None  TranslationStandardOffset=0  TranslationLengthUnit=m  TranslationStandardAxis=+Z  TranslationCartesianOffset=[0 0 0]  TranslationROffset=0  TranslationROffsetUnits=m  TranslationZOffset=0  TranslationZOffsetUnits=m  TranslationThetaOffset=0  TranslationThetaOffsetUnits=deg  RotationMethod=AlignedAxes  RotationAngleUnits=deg  RotationStandardAxis=+Z  RotationAngle=0.0  RotationArbitraryAxis=[0 0 1]  FollAlignAxisA=+Z  BaseAlignAxisA=+Z  FollAlignAxisB=+X  BaseAlignAxisB=+Y  RotationSequenceAxes=FollowerAxes  RotationSequence=XYX  RotationSequenceAngles=[0 0 0]  RotationSequenceAnglesUnits=deg  RotationMatrix=[1 0 0; 0 1 0; 0 0 1]
  Rigid Transform : sm_lib/Frames and Transforms/Rigid Transform  TranslationMethod=Cartesian  TranslationStandardOffset=1  TranslationLengthUnit=m  TranslationStandardAxis=+X  TranslationCartesianOffset="[1  0 0]"  TranslationROffset=0  TranslationROffsetUnits=m  TranslationZOffset=0  TranslationZOffsetUnits=m  TranslationThetaOffset=0  TranslationThetaOffsetUnits=deg  RotationMethod=None  RotationAngleUnits=deg  RotationStandardAxis=+Z  RotationAngle=0  RotationArbitraryAxis=[0 0 1]  FollAlignAxisA=+X  BaseAlignAxisA=+Y  FollAlignAxisB=+Y  BaseAlignAxisB=+Z  RotationSequenceAxes=FollowerAxes  RotationSequence=XYX  RotationSequenceAngles=[0 0 0]  RotationSequenceAnglesUnits=deg  RotationMatrix=[1 0 0; 0 1 0; 0 0 1]
  Scope1 : Scope  NumInputPorts=2
  Simulink-PS Converter{,1..6} (7 alike) : nesl_utility/Simulink-PS Converter  PhysicalDomain=network_engine_domain  SubClassName=ps_input  LeftPortType=input  RightPortType=output  PseudoPeriodic=off  Frequencies=[]  NoiseDistribution=none  NoiseParameters=[]  Unit=N*m  AffineConversion=off  FilteringAndDerivatives=provide  SimscapeFilterOrder=1  InputFilterTimeConstant=0.001  UdotUserProvided=0
  Simulink-PS Converter7 : nesl_utility/Simulink-PS Converter  PhysicalDomain=network_engine_domain  SubClassName=ps_input  LeftPortType=input  RightPortType=output  PseudoPeriodic=off  Frequencies=[]  NoiseDistribution=none  NoiseParameters=[]  Unit=1  AffineConversion=off  FilteringAndDerivatives=provide  SimscapeFilterOrder=1  InputFilterTimeConstant=0.001  UdotUserProvided=0
  Solver Configuration : nesl_utility/Solver Configuration  PhysicalDomain=network_engine_domain  SubClassName=solver  LeftPortType=input  RightPortType=generic  Tones=[]  Harmonics=[]  SimulateNoise=off  Profile=off  UseLocalSampling=off  EnableSwitchedLinearOptims=on  FrequencyDomain=off  UseCCode=off  RelTol=0.001  AbsTol=1e-06  MinStep=1e-09  ToWorkspace=off  RevertToSquareIcSolve=off  NumHomotopyIterations=100  PhasorMode=off  PhasorModeNumHarmonics=1  DoDC=off  ResidualTolerance=1e-09  UseLocalSolver=off  LocalSolverChoice=NE_BACKWARD_EULER_ADVANCER  LocalSolverSampleTime=0.001  DoFixedCost=off  MaxNonlinIter=3  MaxModeIter=2  LinearAlgebra=Sparse  EquationFormulation=NE_TIME_EF  DelaysMemoryBudget=1024  AutomaticFiltering=on  FilteringTimeConstant=0.001  PartitionStorageMethod=AS_NEEDED  PartitionMemoryBudget=1024  PartitionMethod=FAST
  TO: X-forward Y-up Z-lateral : sm_lib/Frames and Transforms/Rigid Transform  TranslationMethod=StandardAxis  TranslationStandardOffset=hatLeftHipToCenterDistWidth/2  TranslationLengthUnit=m  TranslationStandardAxis=+Z  TranslationCartesianOffset=[0 0 0]  TranslationROffset=0  TranslationROffsetUnits=m  TranslationZOffset=0  TranslationZOffsetUnits=m  TranslationThetaOffset=0  TranslationThetaOffsetUnits=deg  RotationMethod=AlignedAxes  RotationAngleUnits=deg  RotationStandardAxis=+Z  RotationAngle=0  RotationArbitraryAxis=[0 0 1]  FollAlignAxisA=+Z  BaseAlignAxisA=+Y  FollAlignAxisB=+X  BaseAlignAxisB=+X  RotationSequenceAxes=FollowerAxes  RotationSequence=XYX  RotationSequenceAngles=[0 0 0]  RotationSequenceAnglesUnits=deg  RotationMatrix=[1 0 0; 0 1 0; 0 0 1]
  World Frame X-forward Y-lateral Z-up1 : sm_lib/Frames and Transforms/World Frame
  body pitch/roll/yaw in body frame --- x-axis: forward y-axis: leftward z-axis: parallel to gravity : Subsystem
  tag scope: HATPosVel=global, LAnklePos=global, LGRF=global, LHipPosVel=global, LKneePos=global, LLBallCnt=global, LLHeelCnt=global, LLLoad=global, LMBallCnt=global, LMHeelCnt=global, LShankPos=global, LphiANDdphiAnkle=global, LphiANDdphiHip=global, LphiANDdphiKnee=global, LthetaANDdthetaHipR=global, RAnklePos=global, RGRF=global, RHipPosVel=global, RKneePos=global, RLBallCnt=global, RLHeelCnt=global, RLLoad=global, RMBallCnt=global, RMHeelCnt=global, RShankPos=global, RphiANDdphiAnkle=global, RphiANDdphiHip=global, RphiANDdphiKnee=global, RthetaANDdthetaHipR=global, front_dv_L=global, front_dv_R=global, leftLegState=global, phiANDdphiHAT=global, psiHAT=global, rightLegState=global, side_dv_L=global, side_dv_R=global, thetaANDdthetaHAT=global
  wires:
  LLHeel Cnt/1 -> L Heel Skin Load Sensor/1
  L Heel Skin Load Sensor/1 -> [LLHeelCnt]
  L Ball Skin Load Sensor/1 -> [LLBallCnt]
  LLBall Cnt/1 -> L Ball Skin Load Sensor/1
  PS-Simulink Converter2/1 -> Mux4/1
  PS-Simulink Converter3/1 -> Mux4/2
  Mux4/1 -> [LphiANDdphiKnee]
  PS-Simulink Converter/1 -> Mux6/1
  PS-Simulink Converter1/1 -> Mux6/2
  Mux6/1 -> [LphiANDdphiAnkle]
  Position Sensor13/1 -> [LAnklePos], Display4/1
  [RAnkleMoment] -> Simulink-PS Converter7/1
  PS-Simulink Converter12/1 -> Mux5/1
  PS-Simulink Converter13/1 -> Mux5/2
  Mux5/1 -> [RphiANDdphiKnee]
  PS-Simulink Converter14/1 -> Mux7/1
  PS-Simulink Converter15/1 -> Mux7/2
  Mux7/1 -> [RphiANDdphiAnkle]
  Position Sensor15/1 -> Display7/1, [RKneePos]
  Position Sensor11/1 -> Display6/1, [RAnklePos]
  [LHipMoment] -> Simulink-PS Converter2/1
  PS-Simulink Converter4/1 -> Mux2/1
  PS-Simulink Converter5/1 -> Mux2/2
  Mux2/1 -> [LphiANDdphiHip]
  PS-Simulink Converter7/1 -> Mux14/2
  PS-Simulink Converter6/1 -> Mux14/1
  Mux14/1 -> [LthetaANDdthetaHipR]
  [LHipMomentR] -> Simulink-PS Converter3/1
  PS-Simulink Converter8/1 -> Mux3/1
  PS-Simulink Converter9/1 -> Mux3/2
  Mux3/1 -> [RphiANDdphiHip]
  Mux15/1 -> L GLU Golgi Tendon Organs3/1
  [RHipMomentR] -> L GLU Golgi Tendon Organs1/1
  L GLU Golgi Tendon Organs3/1 -> [RthetaANDdthetaHipR]
  L GLU Golgi Tendon Organs1/1 -> Simulink-PS Converter5/1
  Position Sensor5/1 -> Display8/1, HAT Position9/1
  Position Sensor6/1 -> HAT Position10/1, Display9/1
  LMHeel Cnt/1 -> L Heel Skin Load Sensor1/1
  L Heel Skin Load Sensor1/1 -> [LMHeelCnt]
  L Ball Skin Load Sensor1/1 -> [LMBallCnt]
  LMBall Cnt/1 -> L Ball Skin Load Sensor1/1
  RLHeel Cnt/1 -> L Heel Skin Load Sensor2/1
  "RMHeel Cnt "/1 -> L Heel Skin Load Sensor3/1
  RMBall Cnt/1 -> L Ball Skin Load Sensor3/1
  RLBall Cnt/1 -> L Ball Skin Load Sensor2/1
  L Heel Skin Load Sensor2/1 -> [RLHeelCnt]
  L Heel Skin Load Sensor3/1 -> [RMHeelCnt]
  L Ball Skin Load Sensor3/1 -> [RMBallCnt]
  L Ball Skin Load Sensor2/1 -> [RLBallCnt]
  Left Thigh/1 -> [LLLoad], Display16/1
  Right Thigh/1 -> [RLLoad], Display18/1
  [RAnklePos] -> "Left lateral d, v in body frame"/2
  [HATPosVel] -> "Right lateral d, v in body frame"/3, "Left lateral d, v in body frame"/3
  [psiHAT] -> "Left lateral d, v in body frame"/1, "Right lateral d, v in body frame"/1
  [LAnklePos] -> "Right lateral d, v in body frame"/2
  "Left lateral d, v in body frame"/1 -> L GLU Golgi Tendon Organs5/1
  [RAnklePos] -> "Left sagittal d, v in body frame"/2
  [HATPosVel] -> "Left sagittal d, v in body frame"/3, "Right sagittal d, v in body frame"/3
  [psiHAT] -> "Right sagittal d, v in body frame"/1, "Left sagittal d, v in body frame"/1
  [LAnklePos] -> "Right sagittal d, v in body frame"/2
  "Left sagittal d, v in body frame"/1 -> [front_dv_L]
  "Right sagittal d, v in body frame"/1 -> [front_dv_R]
  L GLU Golgi Tendon Organs5/1 -> [side_dv_L]
  "Right lateral d, v in body frame"/1 -> [side_dv_R]
  LMHeel Cnt/2 -> Add2/2, Display1/1
  LMBall Cnt/2 -> Add2/3, Display2/1
  LLBall Cnt/2 -> Add2/4, Display3/1
  RLHeel Cnt/2 -> Add1/1, Display27/1
  "RMHeel Cnt "/2 -> Display28/1, Add1/2
  RMBall Cnt/2 -> Add1/3, Display29/1
  RLBall Cnt/2 -> Add1/4, Display30/1
  Position Sensor3/1 -> Display15/1, HAT Position16/1
  Position Sensor2/1 -> Display14/1, HAT Position15/1
  Position Sensor1/1 -> Display13/1, HAT Position18/1
  Position Sensor/1 -> HAT Position17/1, Display12/1
  Position Sensor14/1 -> Display5/1, [LKneePos]
  PS-Simulink Converter10/1 -> Mux15/1
  PS-Simulink Converter11/1 -> Mux15/2
  Position Sensor7/1 -> Display11/1, HAT Position4/1
  Position Sensor8/1 -> Display10/1, HAT Position3/1
  [LAnkleMoment] -> Simulink-PS Converter/1
  body pitch/roll/yaw in body frame --- x-axis: forward y-axis: leftward z-axis: parallel to gravity/3(yaw) -> [psiHAT]
  LLHeel Cnt/2 -> Display/1, Add2/1
  Position Sensor12/1 -> [LShankPos], Display22/1
  Position Sensor4/1 -> Display23/1
  Position Sensor9/1 -> Display24/1
  Position Sensor10/1 -> Display25/1, [RShankPos]
  [LHipPosVel] -> Detect Gait Phase/3
  [LAnklePos] -> Detect Gait Phase/5
  Detect Gait Phase/1 -> Scope1/1, [leftLegState]  "leftLegState"
  [RAnklePos] -> Detect Gait Phase/6
  [RGRF] -> Detect Gait Phase/2
  [RHipPosVel] -> Detect Gait Phase/4
  [LShankPos] -> Detect Gait Phase/7
  Detect Gait Phase/2 -> Scope1/2, [rightLegState]  "rightLegState"
  [RShankPos] -> Detect Gait Phase/8
  [LGRF] -> Detect Gait Phase/1
  Add1/1 -> [RGRF]
  Add2/1 -> [LGRF]
  Position Velocity Sensor1/1 -> [LHipPosVel]
  Position Velocity Sensor2/1 -> [RHipPosVel]
  Position Velocity Sensor/1 -> [HATPosVel]
  [HATPosVel] -> body pitch/roll/yaw in body frame --- x-axis: forward y-axis: leftward z-axis: parallel to gravity/2(HAT Pos Vel)
  [RHipPosVel] -> body pitch/roll/yaw in body frame --- x-axis: forward y-axis: leftward z-axis: parallel to gravity/3(Right Hip Pos Vel)
  [LHipPosVel] -> body pitch/roll/yaw in body frame --- x-axis: forward y-axis: leftward z-axis: parallel to gravity/1(Left Hip Pos Vel)
  body pitch/roll/yaw in body frame --- x-axis: forward y-axis: leftward z-axis: parallel to gravity/1("pitch, pitch velocity") -> [phiANDdphiHAT]
  body pitch/roll/yaw in body frame --- x-axis: forward y-axis: leftward z-axis: parallel to gravity/2("roll, roll velocity") -> [thetaANDdthetaHAT]
  [RHipMoment] -> Simulink-PS Converter4/1
  [LKneeMoment] -> Simulink-PS Converter1/1
  [RKneeMoment] -> Simulink-PS Converter6/1
  connections:
  Left Foot/LConn4 -- LLBall Cnt/LConn1 -- Position Sensor2/LConn1
  Left Foot/LConn3 -- LMBall Cnt/LConn1 -- Position Sensor3/LConn1
  Left Foot/LConn2 -- LMHeel Cnt/LConn1 -- Position Sensor1/LConn1
  Solver Configuration/RConn1 -- Rigid Transform/LConn1 -- World Frame X-forward Y-lateral Z-up1/RConn1 -- TO: X-forward Y-up Z-lateral/RConn1 -- Mechanism Configuration/RConn1
  Rigid Transform/RConn1 -- Ground1/RConn1
  Bushing Joint/LConn1 -- TO: X-forward Y-up Z-lateral/LConn1
  Left Foot/LConn1 -- LLHeel Cnt/LConn1 -- Position Sensor/LConn1
  Bushing Joint/RConn1 -- Left Foot/LConn5
  Left Foot/RConn1 -- Left Ankle joint/LConn1
  Left Ankle joint/LConn2 -- Simulink-PS Converter/RConn1
  Left Ankle joint/RConn2 -- PS-Simulink Converter/LConn1
  Left Ankle joint/RConn3 -- PS-Simulink Converter1/LConn1
  Left Shank/RConn2 -- Position Sensor13/LConn1 -- Left Ankle joint/RConn1
  Position Sensor14/LConn1 -- Left Knee Joint/RConn1 -- Left Thigh/LConn1
  Simulink-PS Converter1/RConn1 -- Left Knee Joint/LConn2
  PS-Simulink Converter2/LConn1 -- Left Knee Joint/RConn2
  Left Knee Joint/RConn3 -- PS-Simulink Converter3/LConn1
  PS-Simulink Converter4/LConn1 -- Left Hip Joint/RConn2
  PS-Simulink Converter5/LConn1 -- Left Hip Joint/RConn3
  PS-Simulink Converter6/LConn1 -- Left Hip Joint/RConn4
  Simulink-PS Converter2/RConn1 -- Left Hip Joint/LConn2
  Simulink-PS Converter3/RConn1 -- Left Hip Joint/LConn3
  PS-Simulink Converter8/LConn1 -- Right Hip joint/RConn2
  Right Hip joint/RConn3 -- PS-Simulink Converter9/LConn1
  Right Hip joint/RConn4 -- PS-Simulink Converter10/LConn1
  Right Hip joint/RConn5 -- PS-Simulink Converter11/LConn1
  Simulink-PS Converter4/RConn1 -- Right Hip joint/LConn2
  Simulink-PS Converter5/RConn1 -- Right Hip joint/LConn3
  PS-Simulink Converter12/LConn1 -- Right Knee joint/RConn2
  PS-Simulink Converter13/LConn1 -- Right Knee joint/RConn3
  Position Sensor15/LConn1 -- Right Thigh/LConn1 -- Right Knee joint/RConn1
  Right Knee joint/LConn1 -- Right Shank/LConn1
  Position Sensor11/LConn1 -- Right Shank/RConn2 -- Right Ankle Joint/RConn1
  PS-Simulink Converter14/LConn1 -- Right Ankle Joint/RConn2
  PS-Simulink Converter15/LConn1 -- Right Ankle Joint/RConn3
  Simulink-PS Converter7/RConn1 -- Right Ankle Joint/LConn2
  Right Foot/RConn1 -- Right Ankle Joint/LConn1
  RMBall Cnt/LConn1 -- Right Foot/LConn4 -- Position Sensor7/LConn1
  RLBall Cnt/LConn1 -- Right Foot/LConn3 -- Position Sensor8/LConn1
  "RMHeel Cnt "/LConn1 -- Right Foot/LConn1 -- Position Sensor6/LConn1
  Position Sensor5/LConn1 -- Right Foot/LConn2 -- RLHeel Cnt/LConn1
  Right Hip joint/LConn1 -- Right Thigh/RConn1
  Left Shank/LConn1 -- Left Knee Joint/LConn1
  Left Hip Joint/LConn1 -- Left Thigh/RConn1
  HATs/LConn1 -- Left Hip Joint/RConn1 -- Position Velocity Sensor1/LConn1
  HATs/LConn2 -- Right Hip joint/RConn1 -- Position Velocity Sensor2/LConn1
  Simulink-PS Converter6/RConn1 -- Right Knee joint/LConn2
  Left Hip Joint/RConn5 -- PS-Simulink Converter7/LConn1
  HATs/RConn1 -- Position Velocity Sensor/LConn1
  Position Sensor4/LConn1 -- Left Foot/RConn2
  Right Foot/RConn2 -- Position Sensor9/LConn1
  Position Sensor10/LConn1 -- Right Shank/RConn1
  Position Sensor12/LConn1 -- Left Shank/RConn1
